simulink model "DUALGNSS"  (R2023b)
settings: Solver=VariableStepAuto  StartTime=0.0  StopTime=10.0  RelTol=1e-3
settings Model: Creator=lucaerviati  LastModifiedBy=monis
settings OptimizationCC: ReuseModelBlockBuffer=off

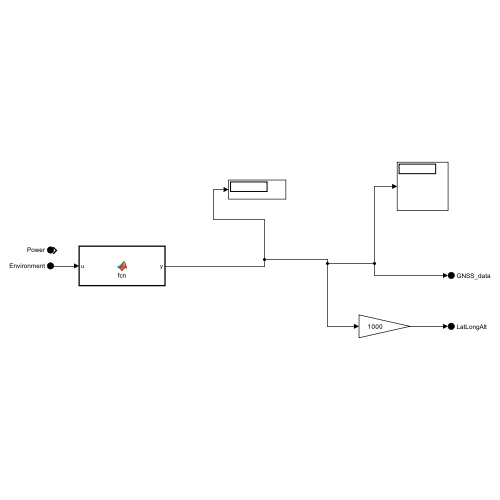
[thumbnail: Simulink's stored preview of the top-level diagram]
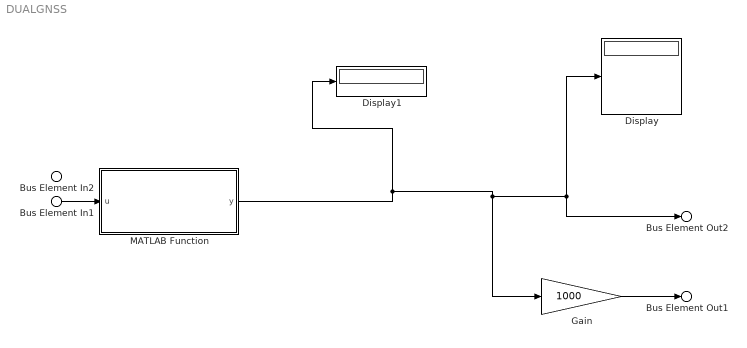
== system DUALGNSS ==
  Bus Element In2 : Inport  PortName=Power
  Bus Element In1 : Inport  Port=2  PortName=Environment
  Display : Display
  Display1 : Display
  Gain : Gain  Gain=1000
  MATLAB Function : MATLAB Function  TreatAsAtomicUnit=on
  Bus Element Out2 : Outport  PortName=GNSS_data
  Bus Element Out1 : Outport  Port=2  PortName=LatLongAlt
  wires:
  MATLAB Function/1(y) -> Display1/1, Gain/1, Display/1, Bus Element Out2/1
  Gain/1 -> Bus Element Out1/1
  Bus Element In1/1 -> MATLAB Function/1(u)

== matlab function DUALGNSS/MATLAB Function ==
  data: u input; y output
function y = fcn(u)
u = [21312,
    12412341,
    12421]
y = u;
